simulink model "simulink_example"  (R2022b)
settings: Solver=VariableStepAuto  StartTime=0.0  StopTime=10.0  RelTol=1e-3
settings Model: Creator=pasho  LastModifiedBy=pasho

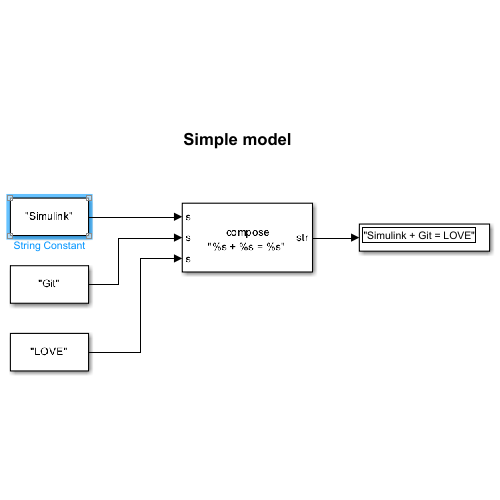
[thumbnail: Simulink's stored preview of the top-level diagram]
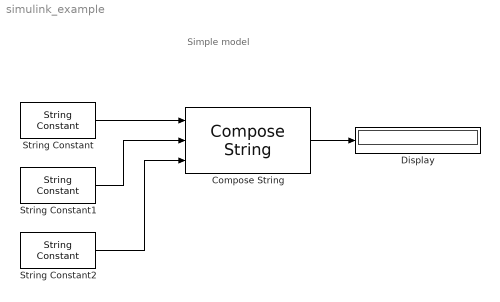
== system simulink_example ==
  note: Simple model
  Compose String : ComposeString  Format="\"%s + %s = %s\""
  Display : Display
  String Constant : StringConstant  String="\"Simulink\""
  String Constant1 : StringConstant  String="\"Git\""
  String Constant2 : StringConstant  String="\"LOVE\""
  wires:
  String Constant/1 -> Compose String/1
  String Constant1/1 -> Compose String/2
  Compose String/1 -> Display/1
  String Constant2/1 -> Compose String/3
